simulink model "ES005A_TmplMonr"  (R2013b)
settings: Solver=ode45  StartTime=0.0  StopTime=2  RelTol=1e-3
values from neighbouring files (symbols this model uses):
  ELECGLBPRM_STRTUPSTTMPLMONININTESTSTRT_CNT_U08 = DataDict.Constant    [ES005A_TmplMonr_DataDict.m]
  IninFlt = DataDict.NTC    [ES005A_TmplMonr_DataDict.m]
  RtFlt = DataDict.NTC    [ES005A_TmplMonr_DataDict.m]
  SpiConf_SpiChannel_TmplMonrCh1 = DataDict.Constant    [ES005A_TmplMonr_DataDict.m]
  SpiConf_SpiChannel_TmplMonrCh2 = DataDict.Constant    [ES005A_TmplMonr_DataDict.m]
  SpiConf_SpiChannel_TmplMonrCh3 = DataDict.Constant    [ES005A_TmplMonr_DataDict.m]
  SpiConf_SpiSequence_TmplMonrSeq1 = DataDict.Constant    [ES005A_TmplMonr_DataDict.m]
  SpiConf_SpiSequence_TmplMonrSeq2 = DataDict.Constant    [ES005A_TmplMonr_DataDict.m]
  SpiConf_SpiSequence_TmplMonrSeq3 = DataDict.Constant    [ES005A_TmplMonr_DataDict.m]
  STD_HIGH = DataDict.Constant    [ES005A_TmplMonr_DataDict.m]
  STD_LOW = DataDict.Constant    [ES005A_TmplMonr_DataDict.m]
  TMPLMONRCFGREG1READVAL_CNT_U16 = DataDict.Constant    [ES005A_TmplMonr_DataDict.m]
  TMPLMONRCFGREG1WRVAL_CNT_U16 = DataDict.Constant    [ES005A_TmplMonr_DataDict.m]
  TMPLMONRSTSREG2READVAL_CNT_U16 = DataDict.Constant    [ES005A_TmplMonr_DataDict.m]
  TMPLMONRWDGMODKEYWORD1_CNT_U16 = DataDict.Constant    [ES005A_TmplMonr_DataDict.m]
  TMPLMONRWDGMODKEYWORD2_CNT_U16 = DataDict.Constant    [ES005A_TmplMonr_DataDict.m]
  TMPLMONRWDGMODKEYWORD3_CNT_U16 = DataDict.Constant    [ES005A_TmplMonr_DataDict.m]
undefined symbols (not defined in the file or in its folder): TrigReg1
libraries: simulink x12
(part 4 of 4)

== system ES005A_TmplMonr/TmplMonr/TmplMonrPer1/TMF Init Test/52/Fault Condition - WD Run Fault/TmplMonrSpiReadWrOrderFlg1 = 1 (Read Buffer)/Spi_ReadIB ==
  note: 00101100
  note: Read Buffer - Simulation Purpose Only
  Channel : Inport
  Constant3 : Constant  Value=44  OutDataTypeStr=uint16
  CopyRight1 : Subsystem  Description=|  mask(Copyright Information){none=on}
      | Copyright info block.                                               
      |                                                                     
      | Place copyright information at the top of every subsystem in design.
      mask prompts: none "No parameters"
      mask help: Place copyright information at the top of every subsystem in design.
      mask Display:
      | NxtrConf = 'Nexteer Confidential';
      | 
      | sys = bdroot; %handle for the current model ("system")
      | first = get_param(sys,'Created');
      | first = first(end-3:end);  %year is last four digits
      | 
      | last = get_param(sys,'LastModifiedDate');
      | if isempty(last)
      |     last = datestr(now,'yyyy');
      | else
      |     last = last(end-3:end);
      | end
      | 
      | if strcmp(first,last)
      |     fprintf('%s -- Copyright %s Nexteer',NxtrConf,first)
      | else
      |     fprintf('%s -- %s%s- %s Nexteer',NxtrConf,char(169),first,last)
      | end
  Terminator : Terminator
  Rx : Outport
  wires:
  Constant3/1 -> Rx/1
  Channel/1 -> Terminator/1

== system ES005A_TmplMonr/TmplMonr/TmplMonrPer1/TMF Init Test/52/Fault Condition - WD Run Fault/TmplMonrSpiReadWrOrderFlg1 = 1 (Read Buffer)/WD_STATE = NOT Watchdog (~=7) ==
  note: NTCNR_0X040
      | Parameters:
      |     1 = 0000 0001 = Bit 0 = Fault Occured Between TmplMonrInitCntr =  9 ~ 10
      |     2 = 0000 0010 = Bit 1 = Fault Occured Between TmplMonrInitCntr = 12 (AND Gate Fault)
      |     4 = 0000 0100 = Bit 2 = Fault Occured Between TmplMonrInitCntr = 14 ~ 15
      |     8 = 0000 1000 = Bit 3 = Fault Occured at TmplMonrInitCntr            = 17  (POE Fault)
      |   16 = 0001 0000 = Bit 4 = Fault Occured at TmplMonrInitCntr            = 18 (WD_STATE Fault)
      |   32 = 0010 0000 = Bit 5 = Fault Occured at TmplMonrInitCntr            = 20 (Edge/Valid Write Fault)
      |   64 = 0100 0000 = Bit 6 = Fault Occured at TmplMonrInitCntr            = 52 (POE + Non-WD Fault)
      | 128 = 1000 0000 = Bit 7 = Fault Occured at TmplMonrInitCntr            = 52 (POE + WD Fault)
  Action Port : ActionPort  ActionType=then
  CopyRight1 : Subsystem  Description=|  mask(Copyright Information){none=on}
      | Copyright info block.                                               
      |                                                                     
      | Place copyright information at the top of every subsystem in design.
      mask prompts: none "No parameters"
      mask help: Place copyright information at the top of every subsystem in design.
      mask Display:
      | NxtrConf = 'Nexteer Confidential';
      | 
      | sys = bdroot; %handle for the current model ("system")
      | first = get_param(sys,'Created');
      | first = first(end-3:end);  %year is last four digits
      | 
      | last = get_param(sys,'LastModifiedDate');
      | if isempty(last)
      |     last = datestr(now,'yyyy');
      | else
      |     last = last(end-3:end);
      | end
      | 
      | if strcmp(first,last)
      |     fprintf('%s -- Copyright %s Nexteer',NxtrConf,first)
      | else
      |     fprintf('%s -- %s%s- %s Nexteer',NxtrConf,char(169),first,last)
      | end
  NtcStInfo : Constant  Value=64  OutDataTypeStr=uint8
  ParamByte : Outport
  wires:
  NtcStInfo/1 -> ParamByte/1

== system ES005A_TmplMonr/TmplMonr/TmplMonrPer1/TMF Init Test/52/Fault Condition - WD Run Fault/TmplMonrSpiReadWrOrderFlg1 = 1 (Read Buffer)/WD_STATE = Watchdog (7) ==
  note: NTCNR_0X040
      | Parameters:
      |     1 = 0000 0001 = Bit 0 = Fault Occured Between TmplMonrInitCntr =  9 ~ 10
      |     2 = 0000 0010 = Bit 1 = Fault Occured Between TmplMonrInitCntr = 12 (AND Gate Fault)
      |     4 = 0000 0100 = Bit 2 = Fault Occured Between TmplMonrInitCntr = 14 ~ 15
      |     8 = 0000 1000 = Bit 3 = Fault Occured at TmplMonrInitCntr            = 17  (POE Fault)
      |   16 = 0001 0000 = Bit 4 = Fault Occured at TmplMonrInitCntr            = 18 (WD_STATE Fault)
      |   32 = 0010 0000 = Bit 5 = Fault Occured at TmplMonrInitCntr            = 20 (Edge/Valid Write Fault)
      |   64 = 0100 0000 = Bit 6 = Fault Occured at TmplMonrInitCntr            = 52 (POE + Non-WD Fault)
      | 128 = 1000 0000 = Bit 7 = Fault Occured at TmplMonrInitCntr            = 52 (POE + WD Fault)
  Action Port : ActionPort  ActionType=else
  CopyRight1 : Subsystem  Description=|  mask(Copyright Information){none=on}
      | Copyright info block.                                               
      |                                                                     
      | Place copyright information at the top of every subsystem in design.
      mask prompts: none "No parameters"
      mask help: Place copyright information at the top of every subsystem in design.
      mask Display:
      | NxtrConf = 'Nexteer Confidential';
      | 
      | sys = bdroot; %handle for the current model ("system")
      | first = get_param(sys,'Created');
      | first = first(end-3:end);  %year is last four digits
      | 
      | last = get_param(sys,'LastModifiedDate');
      | if isempty(last)
      |     last = datestr(now,'yyyy');
      | else
      |     last = last(end-3:end);
      | end
      | 
      | if strcmp(first,last)
      |     fprintf('%s -- Copyright %s Nexteer',NxtrConf,first)
      | else
      |     fprintf('%s -- %s%s- %s Nexteer',NxtrConf,char(169),first,last)
      | end
  NtcStInfo : Constant  Value=128  OutDataTypeStr=uint8
  ParamByte : Outport
  wires:
  NtcStInfo/1 -> ParamByte/1

== system ES005A_TmplMonr/TmplMonr/TmplMonrPer1/TMF Init Test/52/Set NTC 0x040 Note: Run last/FAILED = 1/CopyRight1 ==

== system ES005A_TmplMonr/TmplMonr/TmplMonrPer1/TMF Init Test/52/Set NTC 0x040 Note: Run last/FAILED = 1/SetNtcSts ==
  note: Note:
      |
      | - "ISO Fault Debounce Design" Simulink block intent to use here for Simulation purpose only. Do not Code this block
  NtcNr : Inport
  NtcStInfo : Inport  Port=2
  NtcSts : Inport  Port=3  OutDataTypeStr=uint8
  DebStep : Inport  Port=4  OutDataTypeStr=uint16
  CopyRight2 : Subsystem  Description=|  mask(Copyright Information){none=on}
      | Copyright info block.                                               
      |                                                                     
      | Place copyright information at the top of every subsystem in design.
      mask prompts: none "No parameters"
      mask help: Place copyright information at the top of every subsystem in design.
      mask Display:
      | NxtrConf = 'Nexteer Confidential';
      | 
      | sys = bdroot; %handle for the current model ("system")
      | first = get_param(sys,'Created');
      | first = first(end-3:end);  %year is last four digits
      | 
      | last = get_param(sys,'LastModifiedDate');
      | if isempty(last)
      |     last = datestr(now,'yyyy');
      | else
      |     last = last(end-3:end);
      | end
      | 
      | if strcmp(first,last)
      |     fprintf('%s -- Copyright %s Nexteer',NxtrConf,first)
      | else
      |     fprintf('%s -- %s%s- %s Nexteer',NxtrConf,char(169),first,last)
      | end
  Ground : Ground
  ISO Fault Debounce Design : Stateflow chart  TreatAsAtomicUnit=on
      settings: AttributesFormatString=|
      | Simulation Purpose Only.
      | Do Not Code this block
      | Diagnostic Manager Owns this requirement
  Scope1 : Scope  NumInputPorts=3
      settings: YMin=-5~-5~-5  YMax=5~5~5  SaveName=ScopeData5
  Terminator : Terminator
  Terminator1 : Terminator
  wires:
  NtcStInfo/1 -> Terminator1/1
  NtcNr/1 -> Terminator/1
  NtcSts/1 -> ISO Fault Debounce Design/1(NtcSts), Scope1/1
  DebStep/1 -> ISO Fault Debounce Design/2(DebStep), Scope1/2
  ISO Fault Debounce Design/1(Qualifier) -> Scope1/3
  Ground/1 -> ISO Fault Debounce Design/3(SvcClr)

== system ES005A_TmplMonr/TmplMonr/TmplMonrPer1/TMF Init Test/52/Set NTC 0x040 Note: Run last/PASSED = 0/CopyRight1 ==

== system ES005A_TmplMonr/TmplMonr/TmplMonrPer1/TMF Init Test/52/Set NTC 0x040 Note: Run last/PASSED = 0/SetNtcSts ==
  note: Note:
      |
      | - "ISO Fault Debounce Design" Simulink block intent to use here for Simulation purpose only. Do not Code this block
  NtcNr : Inport
  NtcStInfo : Inport  Port=2
  NtcSts : Inport  Port=3  OutDataTypeStr=uint8
  DebStep : Inport  Port=4  OutDataTypeStr=uint16
  CopyRight2 : Subsystem  Description=|  mask(Copyright Information){none=on}
      | Copyright info block.                                               
      |                                                                     
      | Place copyright information at the top of every subsystem in design.
      mask prompts: none "No parameters"
      mask help: Place copyright information at the top of every subsystem in design.
      mask Display:
      | NxtrConf = 'Nexteer Confidential';
      | 
      | sys = bdroot; %handle for the current model ("system")
      | first = get_param(sys,'Created');
      | first = first(end-3:end);  %year is last four digits
      | 
      | last = get_param(sys,'LastModifiedDate');
      | if isempty(last)
      |     last = datestr(now,'yyyy');
      | else
      |     last = last(end-3:end);
      | end
      | 
      | if strcmp(first,last)
      |     fprintf('%s -- Copyright %s Nexteer',NxtrConf,first)
      | else
      |     fprintf('%s -- %s%s- %s Nexteer',NxtrConf,char(169),first,last)
      | end
  Ground : Ground
  ISO Fault Debounce Design : Stateflow chart  TreatAsAtomicUnit=on
      settings: AttributesFormatString=|
      | Simulation Purpose Only.
      | Do Not Code this block
      | Diagnostic Manager Owns this requirement
  Scope1 : Scope  NumInputPorts=3
      settings: YMin=-5~-5~-5  YMax=5~5~5  SaveName=ScopeData5
  Terminator : Terminator
  Terminator1 : Terminator
  wires:
  NtcStInfo/1 -> Terminator1/1
  NtcNr/1 -> Terminator/1
  NtcSts/1 -> ISO Fault Debounce Design/1(NtcSts), Scope1/1
  DebStep/1 -> ISO Fault Debounce Design/2(DebStep), Scope1/2
  ISO Fault Debounce Design/1(Qualifier) -> Scope1/3
  Ground/1 -> ISO Fault Debounce Design/3(SvcClr)

== system ES005A_TmplMonr/TmplMonr/TmplMonrPer1/TMF Init Test/9-10, 14-16/IoHwAb_GetGpioPwrOutpEnaFb1/Fault Condition - WD Signal/CopyRight1 ==

== system ES005A_TmplMonr/TmplMonr/TmplMonrPer1/TMF Init Test/9-10, 14-16/IoHwAb_GetGpioPwrOutpEnaFb1/IoHwAb_GetGpioPwrOutpEnaFb/CopyRight1 ==

== system ES005A_TmplMonr/TmplMonr/TmplMonrPer1/TMF Run/Fault Condition - WD Run Fault/TmplMonrSpiReadWrOrderFlg2 = 0 (Read Cmd) /Call_Spi_AsyncTransmit/CopyRight1 ==

== system ES005A_TmplMonr/TmplMonr/TmplMonrPer1/TMF Run/Fault Condition - WD Run Fault/TmplMonrSpiReadWrOrderFlg2 = 0 (Read Cmd) /Spi_WriteIB/CopyRight1 ==

== system ES005A_TmplMonr/TmplMonr/TmplMonrPer1/TMF Run/Fault Condition - WD Run Fault/TmplMonrSpiReadWrOrderFlg2 = 1 (Read Buffer)/Spi_ReadIB/CopyRight1 ==

== system ES005A_TmplMonr/TmplMonr/TmplMonrPer1/TMF Run/Fault Condition - WD Run Fault/TmplMonrSpiReadWrOrderFlg2 = 1 (Read Buffer)/WD_STATE = NOT Watchdog (~7)/CopyRight1 ==

== system ES005A_TmplMonr/TmplMonr/TmplMonrPer1/TMF Run/Fault Condition - WD Run Fault/TmplMonrSpiReadWrOrderFlg2 = 1 (Read Buffer)/WD_STATE = NOT Watchdog (~7)/SetNtcSts ==
  note: Note:
      |
      | - "ISO Fault Debounce Design" Simulink block intent to use here for Simulation purpose only. Do not Code this block
  NtcNr : Inport
  NtcStInfo : Inport  Port=2
  NtcSts : Inport  Port=3  OutDataTypeStr=uint8
  DebStep : Inport  Port=4  OutDataTypeStr=uint16
  CopyRight2 : Subsystem  Description=|  mask(Copyright Information){none=on}
      | Copyright info block.                                               
      |                                                                     
      | Place copyright information at the top of every subsystem in design.
      mask prompts: none "No parameters"
      mask help: Place copyright information at the top of every subsystem in design.
      mask Display:
      | NxtrConf = 'Nexteer Confidential';
      | 
      | sys = bdroot; %handle for the current model ("system")
      | first = get_param(sys,'Created');
      | first = first(end-3:end);  %year is last four digits
      | 
      | last = get_param(sys,'LastModifiedDate');
      | if isempty(last)
      |     last = datestr(now,'yyyy');
      | else
      |     last = last(end-3:end);
      | end
      | 
      | if strcmp(first,last)
      |     fprintf('%s -- Copyright %s Nexteer',NxtrConf,first)
      | else
      |     fprintf('%s -- %s%s- %s Nexteer',NxtrConf,char(169),first,last)
      | end
  Ground : Ground
  ISO Fault Debounce Design : Stateflow chart  TreatAsAtomicUnit=on
      settings: AttributesFormatString=|
      | Simulation Purpose Only.
      | Do Not Code this block
      | Diagnostic Manager Owns this requirement
  Scope1 : Scope  NumInputPorts=3
      settings: YMin=-5~-5~-5  YMax=5~5~5  SaveName=ScopeData5
  Terminator : Terminator
  Terminator1 : Terminator
  wires:
  NtcStInfo/1 -> Terminator1/1
  NtcNr/1 -> Terminator/1
  NtcSts/1 -> ISO Fault Debounce Design/1(NtcSts), Scope1/1
  DebStep/1 -> ISO Fault Debounce Design/2(DebStep), Scope1/2
  ISO Fault Debounce Design/1(Qualifier) -> Scope1/3
  Ground/1 -> ISO Fault Debounce Design/3(SvcClr)

== system ES005A_TmplMonr/TmplMonr/TmplMonrPer1/TMF Run/Fault Condition - WD Run Fault/TmplMonrSpiReadWrOrderFlg2 = 1 (Read Buffer)/WD_STATE = Watchdog (7)/CopyRight1 ==

== system ES005A_TmplMonr/TmplMonr/TmplMonrPer1/TMF Run/Fault Condition - WD Run Fault/TmplMonrSpiReadWrOrderFlg2 = 1 (Read Buffer)/WD_STATE = Watchdog (7)/SetNtcSts ==
  note: Note:
      |
      | - "ISO Fault Debounce Design" Simulink block intent to use here for Simulation purpose only. Do not Code this block
  NtcNr : Inport
  NtcStInfo : Inport  Port=2
  NtcSts : Inport  Port=3  OutDataTypeStr=uint8
  DebStep : Inport  Port=4
  CopyRight2 : Subsystem  Description=|  mask(Copyright Information){none=on}
      | Copyright info block.                                               
      |                                                                     
      | Place copyright information at the top of every subsystem in design.
      mask prompts: none "No parameters"
      mask help: Place copyright information at the top of every subsystem in design.
      mask Display:
      | NxtrConf = 'Nexteer Confidential';
      | 
      | sys = bdroot; %handle for the current model ("system")
      | first = get_param(sys,'Created');
      | first = first(end-3:end);  %year is last four digits
      | 
      | last = get_param(sys,'LastModifiedDate');
      | if isempty(last)
      |     last = datestr(now,'yyyy');
      | else
      |     last = last(end-3:end);
      | end
      | 
      | if strcmp(first,last)
      |     fprintf('%s -- Copyright %s Nexteer',NxtrConf,first)
      | else
      |     fprintf('%s -- %s%s- %s Nexteer',NxtrConf,char(169),first,last)
      | end
  Ground : Ground
  ISO Fault Debounce Design : Stateflow chart  TreatAsAtomicUnit=on
      settings: AttributesFormatString=|
      | Simulation Purpose Only.
      | Do Not Code this block
      | Diagnostic Manager Owns this requirement
  Scope1 : Scope  NumInputPorts=3
      settings: YMin=-5~-5~-5  YMax=5~5~5  SaveName=ScopeData5
  Terminator : Terminator
  Terminator1 : Terminator
  wires:
  NtcStInfo/1 -> Terminator1/1
  NtcNr/1 -> Terminator/1
  NtcSts/1 -> ISO Fault Debounce Design/1(NtcSts), Scope1/1
  DebStep/1 -> ISO Fault Debounce Design/2(DebStep), Scope1/2
  ISO Fault Debounce Design/1(Qualifier) -> Scope1/3
  Ground/1 -> ISO Fault Debounce Design/3(SvcClr)

== system ES005A_TmplMonr/TmplMonr/TmplMonrPer1/TMF Init Test/18/WD_STATE = 0 ~ 2, 7/WD RESTART - Two Re-try/Watchdog Mode Key: Word1/Call_Spi_AsyncTransmit ==
  Sequence : Inport
  CopyRight1 : Subsystem  Description=|  mask(Copyright Information){none=on}
      | Copyright info block.                                               
      |                                                                     
      | Place copyright information at the top of every subsystem in design.
      mask prompts: none "No parameters"
      mask help: Place copyright information at the top of every subsystem in design.
      mask Display:
      | NxtrConf = 'Nexteer Confidential';
      | 
      | sys = bdroot; %handle for the current model ("system")
      | first = get_param(sys,'Created');
      | first = first(end-3:end);  %year is last four digits
      | 
      | last = get_param(sys,'LastModifiedDate');
      | if isempty(last)
      |     last = datestr(now,'yyyy');
      | else
      |     last = last(end-3:end);
      | end
      | 
      | if strcmp(first,last)
      |     fprintf('%s -- Copyright %s Nexteer',NxtrConf,first)
      | else
      |     fprintf('%s -- %s%s- %s Nexteer',NxtrConf,char(169),first,last)
      | end
  Terminator : Terminator
  wires:
  Sequence/1 -> Terminator/1

== system ES005A_TmplMonr/TmplMonr/TmplMonrPer1/TMF Init Test/18/WD_STATE = 0 ~ 2, 7/WD RESTART - Two Re-try/Watchdog Mode Key: Word1/CopyRight1 ==

== system ES005A_TmplMonr/TmplMonr/TmplMonrPer1/TMF Init Test/18/WD_STATE = 0 ~ 2, 7/WD RESTART - Two Re-try/Watchdog Mode Key: Word1/Spi_WriteIB ==
  Channel : Inport
  DataBufferPtr : Inport  Port=2
  CopyRight1 : Subsystem  Description=|  mask(Copyright Information){none=on}
      | Copyright info block.                                               
      |                                                                     
      | Place copyright information at the top of every subsystem in design.
      mask prompts: none "No parameters"
      mask help: Place copyright information at the top of every subsystem in design.
      mask Display:
      | NxtrConf = 'Nexteer Confidential';
      | 
      | sys = bdroot; %handle for the current model ("system")
      | first = get_param(sys,'Created');
      | first = first(end-3:end);  %year is last four digits
      | 
      | last = get_param(sys,'LastModifiedDate');
      | if isempty(last)
      |     last = datestr(now,'yyyy');
      | else
      |     last = last(end-3:end);
      | end
      | 
      | if strcmp(first,last)
      |     fprintf('%s -- Copyright %s Nexteer',NxtrConf,first)
      | else
      |     fprintf('%s -- %s%s- %s Nexteer',NxtrConf,char(169),first,last)
      | end
  Terminator : Terminator
  Terminator1 : Terminator
  wires:
  Channel/1 -> Terminator/1
  DataBufferPtr/1 -> Terminator1/1

== system ES005A_TmplMonr/TmplMonr/TmplMonrPer1/TMF Init Test/18/WD_STATE = 0 ~ 2, 7/WD RESTART - Two Re-try/Watchdog Mode Key: Word2/Call_Spi_AsyncTransmit ==
  Sequence : Inport
  CopyRight1 : Subsystem  Description=|  mask(Copyright Information){none=on}
      | Copyright info block.                                               
      |                                                                     
      | Place copyright information at the top of every subsystem in design.
      mask prompts: none "No parameters"
      mask help: Place copyright information at the top of every subsystem in design.
      mask Display:
      | NxtrConf = 'Nexteer Confidential';
      | 
      | sys = bdroot; %handle for the current model ("system")
      | first = get_param(sys,'Created');
      | first = first(end-3:end);  %year is last four digits
      | 
      | last = get_param(sys,'LastModifiedDate');
      | if isempty(last)
      |     last = datestr(now,'yyyy');
      | else
      |     last = last(end-3:end);
      | end
      | 
      | if strcmp(first,last)
      |     fprintf('%s -- Copyright %s Nexteer',NxtrConf,first)
      | else
      |     fprintf('%s -- %s%s- %s Nexteer',NxtrConf,char(169),first,last)
      | end
  Terminator : Terminator
  wires:
  Sequence/1 -> Terminator/1

== system ES005A_TmplMonr/TmplMonr/TmplMonrPer1/TMF Init Test/18/WD_STATE = 0 ~ 2, 7/WD RESTART - Two Re-try/Watchdog Mode Key: Word2/CopyRight1 ==

== system ES005A_TmplMonr/TmplMonr/TmplMonrPer1/TMF Init Test/18/WD_STATE = 0 ~ 2, 7/WD RESTART - Two Re-try/Watchdog Mode Key: Word2/Spi_WriteIB ==
  Channel : Inport
  DataBufferPtr : Inport  Port=2
  CopyRight1 : Subsystem  Description=|  mask(Copyright Information){none=on}
      | Copyright info block.                                               
      |                                                                     
      | Place copyright information at the top of every subsystem in design.
      mask prompts: none "No parameters"
      mask help: Place copyright information at the top of every subsystem in design.
      mask Display:
      | NxtrConf = 'Nexteer Confidential';
      | 
      | sys = bdroot; %handle for the current model ("system")
      | first = get_param(sys,'Created');
      | first = first(end-3:end);  %year is last four digits
      | 
      | last = get_param(sys,'LastModifiedDate');
      | if isempty(last)
      |     last = datestr(now,'yyyy');
      | else
      |     last = last(end-3:end);
      | end
      | 
      | if strcmp(first,last)
      |     fprintf('%s -- Copyright %s Nexteer',NxtrConf,first)
      | else
      |     fprintf('%s -- %s%s- %s Nexteer',NxtrConf,char(169),first,last)
      | end
  Terminator : Terminator
  Terminator1 : Terminator
  wires:
  Channel/1 -> Terminator/1
  DataBufferPtr/1 -> Terminator1/1

== system ES005A_TmplMonr/TmplMonr/TmplMonrPer1/TMF Init Test/18/WD_STATE = 0 ~ 2, 7/WD RESTART - Two Re-try/Watchdog Mode Key: Word3/Call_Spi_AsyncTransmit ==
  Sequence : Inport
  CopyRight1 : Subsystem  Description=|  mask(Copyright Information){none=on}
      | Copyright info block.                                               
      |                                                                     
      | Place copyright information at the top of every subsystem in design.
      mask prompts: none "No parameters"
      mask help: Place copyright information at the top of every subsystem in design.
      mask Display:
      | NxtrConf = 'Nexteer Confidential';
      | 
      | sys = bdroot; %handle for the current model ("system")
      | first = get_param(sys,'Created');
      | first = first(end-3:end);  %year is last four digits
      | 
      | last = get_param(sys,'LastModifiedDate');
      | if isempty(last)
      |     last = datestr(now,'yyyy');
      | else
      |     last = last(end-3:end);
      | end
      | 
      | if strcmp(first,last)
      |     fprintf('%s -- Copyright %s Nexteer',NxtrConf,first)
      | else
      |     fprintf('%s -- %s%s- %s Nexteer',NxtrConf,char(169),first,last)
      | end
  Terminator : Terminator
  wires:
  Sequence/1 -> Terminator/1

== system ES005A_TmplMonr/TmplMonr/TmplMonrPer1/TMF Init Test/18/WD_STATE = 0 ~ 2, 7/WD RESTART - Two Re-try/Watchdog Mode Key: Word3/CopyRight1 ==

== system ES005A_TmplMonr/TmplMonr/TmplMonrPer1/TMF Init Test/18/WD_STATE = 0 ~ 2, 7/WD RESTART - Two Re-try/Watchdog Mode Key: Word3/Spi_WriteIB ==
  Channel : Inport
  DataBufferPtr : Inport  Port=2
  CopyRight1 : Subsystem  Description=|  mask(Copyright Information){none=on}
      | Copyright info block.                                               
      |                                                                     
      | Place copyright information at the top of every subsystem in design.
      mask prompts: none "No parameters"
      mask help: Place copyright information at the top of every subsystem in design.
      mask Display:
      | NxtrConf = 'Nexteer Confidential';
      | 
      | sys = bdroot; %handle for the current model ("system")
      | first = get_param(sys,'Created');
      | first = first(end-3:end);  %year is last four digits
      | 
      | last = get_param(sys,'LastModifiedDate');
      | if isempty(last)
      |     last = datestr(now,'yyyy');
      | else
      |     last = last(end-3:end);
      | end
      | 
      | if strcmp(first,last)
      |     fprintf('%s -- Copyright %s Nexteer',NxtrConf,first)
      | else
      |     fprintf('%s -- %s%s- %s Nexteer',NxtrConf,char(169),first,last)
      | end
  Terminator : Terminator
  Terminator1 : Terminator
  wires:
  Channel/1 -> Terminator/1
  DataBufferPtr/1 -> Terminator1/1

== system ES005A_TmplMonr/TmplMonr/TmplMonrPer1/TMF Init Test/52/Fault Condition - WD Run Fault/TmplMonrSpiReadWrOrderFlg1 = 0 (Read Cmd) /Call_Spi_AsyncTransmit/CopyRight1 ==

== system ES005A_TmplMonr/TmplMonr/TmplMonrPer1/TMF Init Test/52/Fault Condition - WD Run Fault/TmplMonrSpiReadWrOrderFlg1 = 0 (Read Cmd) /Spi_WriteIB/CopyRight1 ==

== system ES005A_TmplMonr/TmplMonr/TmplMonrPer1/TMF Init Test/52/Fault Condition - WD Run Fault/TmplMonrSpiReadWrOrderFlg1 = 1 (Read Buffer)/Spi_ReadIB/CopyRight1 ==

== system ES005A_TmplMonr/TmplMonr/TmplMonrPer1/TMF Init Test/52/Fault Condition - WD Run Fault/TmplMonrSpiReadWrOrderFlg1 = 1 (Read Buffer)/WD_STATE = NOT Watchdog (~=7)/CopyRight1 ==

== system ES005A_TmplMonr/TmplMonr/TmplMonrPer1/TMF Init Test/52/Fault Condition - WD Run Fault/TmplMonrSpiReadWrOrderFlg1 = 1 (Read Buffer)/WD_STATE = Watchdog (7)/CopyRight1 ==

== system ES005A_TmplMonr/TmplMonr/TmplMonrPer1/TMF Init Test/52/Set NTC 0x040 Note: Run last/FAILED = 1/SetNtcSts/CopyRight2 ==

== system ES005A_TmplMonr/TmplMonr/TmplMonrPer1/TMF Init Test/52/Set NTC 0x040 Note: Run last/PASSED = 0/SetNtcSts/CopyRight2 ==

== system ES005A_TmplMonr/TmplMonr/TmplMonrPer1/TMF Run/Fault Condition - WD Run Fault/TmplMonrSpiReadWrOrderFlg2 = 1 (Read Buffer)/WD_STATE = NOT Watchdog (~7)/SetNtcSts/CopyRight2 ==

== system ES005A_TmplMonr/TmplMonr/TmplMonrPer1/TMF Run/Fault Condition - WD Run Fault/TmplMonrSpiReadWrOrderFlg2 = 1 (Read Buffer)/WD_STATE = Watchdog (7)/SetNtcSts/CopyRight2 ==

== system ES005A_TmplMonr/TmplMonr/TmplMonrPer1/TMF Init Test/18/WD_STATE = 0 ~ 2, 7/WD RESTART - Two Re-try/Watchdog Mode Key: Word1/Call_Spi_AsyncTransmit/CopyRight1 ==

== system ES005A_TmplMonr/TmplMonr/TmplMonrPer1/TMF Init Test/18/WD_STATE = 0 ~ 2, 7/WD RESTART - Two Re-try/Watchdog Mode Key: Word1/Spi_WriteIB/CopyRight1 ==

== system ES005A_TmplMonr/TmplMonr/TmplMonrPer1/TMF Init Test/18/WD_STATE = 0 ~ 2, 7/WD RESTART - Two Re-try/Watchdog Mode Key: Word2/Call_Spi_AsyncTransmit/CopyRight1 ==

== system ES005A_TmplMonr/TmplMonr/TmplMonrPer1/TMF Init Test/18/WD_STATE = 0 ~ 2, 7/WD RESTART - Two Re-try/Watchdog Mode Key: Word2/Spi_WriteIB/CopyRight1 ==

== system ES005A_TmplMonr/TmplMonr/TmplMonrPer1/TMF Init Test/18/WD_STATE = 0 ~ 2, 7/WD RESTART - Two Re-try/Watchdog Mode Key: Word3/Call_Spi_AsyncTransmit/CopyRight1 ==

== system ES005A_TmplMonr/TmplMonr/TmplMonrPer1/TMF Init Test/18/WD_STATE = 0 ~ 2, 7/WD RESTART - Two Re-try/Watchdog Mode Key: Word3/Spi_WriteIB/CopyRight1 ==

== stateflow chart ES005A_TmplMonr/TmplMonr/TmplMonrPer1/TMF Init Test/52/Set NTC 0x040 Note: Run last/PASSED = 0/SetNtcSts/ISO Fault Debounce Design ==
  note: NTCSTS_PASSD           (0)
      | NTCSTS_FAILD             (1)
      | NTCSTS_PREPASSD   (2)
      | NTCSTS_PREFAILD     (3)
      |
      | SIGQLFR_NORES        (0)
      | SIGQLFR_PASSD         (1)
      | SIGQLFR_FAILD           (2)
  note: Pass Loop
  note: Fail Loop
  note: 
  (default) -> (junction 89)
  (junction 89) -> (junction 95) [order 1] : [NtcSts ==3]
  (junction 89) -> (junction 93) [order 2] : [NtcSts ==2]
  (junction 89) -> (junction 141) [order 3] : [NtcSts ==1]
      | { ErrAcc = 32767;
      | Qualifier =2;
      |  }
  (junction 89) -> (junction 141) [order 4] : [NtcSts ==0]
      | { ErrAcc = -32768;
      | Qualifier=1;
      | }
  (junction 95) -> (junction 103) [order 2]
  (junction 95) -> (junction 111) [order 1] : [ErrAcc <=0]
      | {ErrAcc = DebStep;}
  (junction 93) -> (junction 123) [order 2] : {
      | ErrAcc = ErrAcc - DebStep;
      | }
  (junction 93) -> (junction 123) [order 1] : [(ErrAcc - DebStep) <= -32768]
      | { ErrAcc = -32768;
      | Qualifier=1;
      | }
  (junction 103) -> (junction 111) [order 1] : [(ErrAcc + DebStep) <32767]
      | {ErrAcc = ErrAcc + DebStep;}
  (junction 103) -> (junction 111) [order 2] : {ErrAcc = 32767;
      | Qualifier =2;}
  (junction 123) -> (junction 141)
  (junction 111) -> (junction 141)
  (junction 141) -> (junction 159) [order 2] : {ErrAcc = 0;
      | Qualifier =0;
      | }
  (junction 141) -> (junction 159) [order 1] : [SvcClr ==0]
  data: NtcSts input uint8; Qualifier output uint8; DebStep input uint16; ErrAcc local int16; SvcClr input

== stateflow chart ES005A_TmplMonr/TmplMonr/TmplMonrPer1/TMF Run/Fault Condition - WD Run Fault/TmplMonrSpiReadWrOrderFlg2 = 1 (Read Buffer)/WD_STATE = Watchdog (7)/SetNtcSts/ISO Fault Debounce Design ==
  note: NTCSTS_PASSD           (0)
      | NTCSTS_FAILD             (1)
      | NTCSTS_PREPASSD   (2)
      | NTCSTS_PREFAILD     (3)
      |
      | SIGQLFR_NORES        (0)
      | SIGQLFR_PASSD         (1)
      | SIGQLFR_FAILD           (2)
  note: Pass Loop
  note: Fail Loop
  note: 
  (default) -> (junction 89)
  (junction 89) -> (junction 95) [order 1] : [NtcSts ==3]
  (junction 89) -> (junction 93) [order 2] : [NtcSts ==2]
  (junction 89) -> (junction 141) [order 3] : [NtcSts ==1]
      | { ErrAcc = 32767;
      | Qualifier =2;
      |  }
  (junction 89) -> (junction 141) [order 4] : [NtcSts ==0]
      | { ErrAcc = -32768;
      | Qualifier=1;
      | }
  (junction 95) -> (junction 103) [order 2]
  (junction 95) -> (junction 111) [order 1] : [ErrAcc <=0]
      | {ErrAcc = DebStep;}
  (junction 93) -> (junction 123) [order 2] : {
      | ErrAcc = ErrAcc - DebStep;
      | }
  (junction 93) -> (junction 123) [order 1] : [(ErrAcc - DebStep) <= -32768]
      | { ErrAcc = -32768;
      | Qualifier=1;
      | }
  (junction 103) -> (junction 111) [order 1] : [(ErrAcc + DebStep) <32767]
      | {ErrAcc = ErrAcc + DebStep;}
  (junction 103) -> (junction 111) [order 2] : {ErrAcc = 32767;
      | Qualifier =2;}
  (junction 123) -> (junction 141)
  (junction 111) -> (junction 141)
  (junction 141) -> (junction 159) [order 2] : {ErrAcc = 0;
      | Qualifier =0;
      | }
  (junction 141) -> (junction 159) [order 1] : [SvcClr ==0]
  data: NtcSts input uint8; Qualifier output uint8; DebStep input uint16; ErrAcc local int16; SvcClr input

== stateflow chart ES005A_TmplMonr/TmplMonr/TmplMonrPer1/TMF Run/Normal Condition/SetNtcSts/ISO Fault Debounce Design ==
  note: NTCSTS_PASSD           (0)
      | NTCSTS_FAILD             (1)
      | NTCSTS_PREPASSD   (2)
      | NTCSTS_PREFAILD     (3)
      |
      | SIGQLFR_NORES        (0)
      | SIGQLFR_PASSD         (1)
      | SIGQLFR_FAILD           (2)
  note: Pass Loop
  note: Fail Loop
  note: 
  (default) -> (junction 89)
  (junction 89) -> (junction 95) [order 1] : [NtcSts ==3]
  (junction 89) -> (junction 93) [order 2] : [NtcSts ==2]
  (junction 89) -> (junction 141) [order 3] : [NtcSts ==1]
      | { ErrAcc = 32767;
      | Qualifier =2;
      |  }
  (junction 89) -> (junction 141) [order 4] : [NtcSts ==0]
      | { ErrAcc = -32768;
      | Qualifier=1;
      | }
  (junction 95) -> (junction 103) [order 2]
  (junction 95) -> (junction 111) [order 1] : [ErrAcc <=0]
      | {ErrAcc = DebStep;}
  (junction 93) -> (junction 123) [order 2] : {
      | ErrAcc = ErrAcc - DebStep;
      | }
  (junction 93) -> (junction 123) [order 1] : [(ErrAcc - DebStep) <= -32768]
      | { ErrAcc = -32768;
      | Qualifier=1;
      | }
  (junction 103) -> (junction 111) [order 1] : [(ErrAcc + DebStep) <32767]
      | {ErrAcc = ErrAcc + DebStep;}
  (junction 103) -> (junction 111) [order 2] : {ErrAcc = 32767;
      | Qualifier =2;}
  (junction 123) -> (junction 141)
  (junction 111) -> (junction 141)
  (junction 141) -> (junction 159) [order 2] : {ErrAcc = 0;
      | Qualifier =0;
      | }
  (junction 141) -> (junction 159) [order 1] : [SvcClr ==0]
  data: NtcSts input uint8; Qualifier output uint8; DebStep input uint16; ErrAcc local int16; SvcClr input

== stateflow chart ES005A_TmplMonr/TmplMonr/TmplMonrPer1/TMF Run/Fault Condition - WD Run Fault/TmplMonrSpiReadWrOrderFlg2 = 1 (Read Buffer)/WD_STATE = NOT Watchdog (~7)/SetNtcSts/ISO Fault Debounce Design ==
  note: NTCSTS_PASSD           (0)
      | NTCSTS_FAILD             (1)
      | NTCSTS_PREPASSD   (2)
      | NTCSTS_PREFAILD     (3)
      |
      | SIGQLFR_NORES        (0)
      | SIGQLFR_PASSD         (1)
      | SIGQLFR_FAILD           (2)
  note: Pass Loop
  note: Fail Loop
  note: 
  (default) -> (junction 89)
  (junction 89) -> (junction 95) [order 1] : [NtcSts ==3]
  (junction 89) -> (junction 93) [order 2] : [NtcSts ==2]
  (junction 89) -> (junction 141) [order 3] : [NtcSts ==1]
      | { ErrAcc = 32767;
      | Qualifier =2;
      |  }
  (junction 89) -> (junction 141) [order 4] : [NtcSts ==0]
      | { ErrAcc = -32768;
      | Qualifier=1;
      | }
  (junction 95) -> (junction 103) [order 2]
  (junction 95) -> (junction 111) [order 1] : [ErrAcc <=0]
      | {ErrAcc = DebStep;}
  (junction 93) -> (junction 123) [order 2] : {
      | ErrAcc = ErrAcc - DebStep;
      | }
  (junction 93) -> (junction 123) [order 1] : [(ErrAcc - DebStep) <= -32768]
      | { ErrAcc = -32768;
      | Qualifier=1;
      | }
  (junction 103) -> (junction 111) [order 1] : [(ErrAcc + DebStep) <32767]
      | {ErrAcc = ErrAcc + DebStep;}
  (junction 103) -> (junction 111) [order 2] : {ErrAcc = 32767;
      | Qualifier =2;}
  (junction 123) -> (junction 141)
  (junction 111) -> (junction 141)
  (junction 141) -> (junction 159) [order 2] : {ErrAcc = 0;
      | Qualifier =0;
      | }
  (junction 141) -> (junction 159) [order 1] : [SvcClr ==0]
  data: NtcSts input uint8; Qualifier output uint8; DebStep input uint16; ErrAcc local int16; SvcClr input

== stateflow chart ES005A_TmplMonr/TmplMonr/TmplMonrPer1/TMF Init Test/52/Set NTC 0x040 Note: Run last/FAILED = 1/SetNtcSts/ISO Fault Debounce Design ==
  note: NTCSTS_PASSD           (0)
      | NTCSTS_FAILD             (1)
      | NTCSTS_PREPASSD   (2)
      | NTCSTS_PREFAILD     (3)
      |
      | SIGQLFR_NORES        (0)
      | SIGQLFR_PASSD         (1)
      | SIGQLFR_FAILD           (2)
  note: Pass Loop
  note: Fail Loop
  note: 
  (default) -> (junction 89)
  (junction 89) -> (junction 95) [order 1] : [NtcSts ==3]
  (junction 89) -> (junction 93) [order 2] : [NtcSts ==2]
  (junction 89) -> (junction 141) [order 3] : [NtcSts ==1]
      | { ErrAcc = 32767;
      | Qualifier =2;
      |  }
  (junction 89) -> (junction 141) [order 4] : [NtcSts ==0]
      | { ErrAcc = -32768;
      | Qualifier=1;
      | }
  (junction 95) -> (junction 103) [order 2]
  (junction 95) -> (junction 111) [order 1] : [ErrAcc <=0]
      | {ErrAcc = DebStep;}
  (junction 93) -> (junction 123) [order 2] : {
      | ErrAcc = ErrAcc - DebStep;
      | }
  (junction 93) -> (junction 123) [order 1] : [(ErrAcc - DebStep) <= -32768]
      | { ErrAcc = -32768;
      | Qualifier=1;
      | }
  (junction 103) -> (junction 111) [order 1] : [(ErrAcc + DebStep) <32767]
      | {ErrAcc = ErrAcc + DebStep;}
  (junction 103) -> (junction 111) [order 2] : {ErrAcc = 32767;
      | Qualifier =2;}
  (junction 123) -> (junction 141)
  (junction 111) -> (junction 141)
  (junction 141) -> (junction 159) [order 2] : {ErrAcc = 0;
      | Qualifier =0;
      | }
  (junction 141) -> (junction 159) [order 1] : [SvcClr ==0]
  data: NtcSts input uint8; Qualifier output uint8; DebStep input uint16; ErrAcc local int16; SvcClr input
